simulink library "nexys2iroobo_lib"  (Simulink 7.9)
settings: Solver=ode45  StartTime=0.0  StopTime=10.0  RelTol=1e-3
libraries: xbsIndex_r4 x5
settings Model: Creator=gaborsz  LastModifiedBy=gaborsz

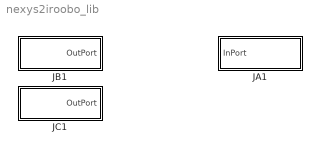
== system nexys2iroobo_lib ==
  JA1 : Subsystem  mask(Non-Memory-Mapped Output Port){show_out=off}
      mask prompts: show_out "Provide Output Double"
      mask help:
      | Port Name: "JA1"
      | Port Type: 8-bit Vector
      mask init:
      | [bg,fg] = xlcmap('IO',0);
      | iPos = get_param(gcb,'Position');
      | iWidth=iPos(3)-iPos(1);
      | iHeight=iPos(4)-iPos(2);
      | [logoX, logoY] = xlogo(iPos);
      | if (show_out)
      |     old = find_system(gcb, 'LookUnderMasks', 'all', 'Name', 'Terminator');
      |     if (length(old) > 0)
      |         replace_block(gcb, 'Name', 'Terminator', 'OutPort', 'noprompt');
      |         set_param([gcb '/Terminator'], 'Name', 'OutPort');
      |     end
      |     portdir = 'output';
      |     portstr = 'dbl';
      | else
      |     old = find_system(gcb, 'LookUnderMasks', 'all', 'name', 'OutPort');
      |     if (length(old) > 0)
      |         replace_block(gcb, 'Name', 'OutPort', 'Terminator', 'noprompt');
      |         set_param([gcb '/OutPort'], 'Name', 'Terminator');
      |     end
      |     portdir = 'input';
      |     portstr = '';
      | end
      settings: CopyFcn=set_param(gcb,'LinkStatus','inactive');
      mask Display:
      | patch([0 iWidth iWidth 0],[0 0 iHeight iHeight] , bg);
      | patch(logoX,logoY, fg);
      | plot([0 0 iWidth iWidth 0], [0 iHeight iHeight 0 0]);
      | port_label(portdir,1,portstr);
      | port_label('input',1,'JA1');
      | text(iWidth-10,5,'nmm');
  JB1 : Subsystem  mask(Non-Memory-Mapped Input Port){signed=off, bpt=0, show_in=off, c=0}
      mask prompts: signed "Signed  (2's comp)"; bpt "Binary Point"; show_in "Provide Input Double"; c "Constant for Simulation"
      mask help:
      | Port Name: "JB1"
      | Port Type: 8-bit Vector
      mask init:
      | [bg,fg] = xlcmap('IO',0);
      | iPos = get_param(gcb,'Position');
      | iWidth=iPos(3)-iPos(1);
      | iHeight=iPos(4)-iPos(2);
      | [logoX, logoY] = xlogo(iPos);
      | if (signed)
      |     set_param([gcb '/JB1'],'arith_type','Signed  (2''s comp)');
      | else
      |     set_param([gcb '/JB1'],'arith_type','Unsigned');
      | end
      | if (show_in)
      |     old = find_system(gcb, 'LookUnderMasks', 'all', 'Name', 'Constant');
      |     if (length(old) > 0)
      |         replace_block(gcb, 'Name', 'Constant', 'InPort', 'noprompt');
      |         set_param([gcb '/Constant'], 'Name', 'InPort');
      |     end
      |     portdir = 'input';
      |     portstr = 'dbl';
      | else
      |     old = find_system(gcb, 'LookUnderMasks', 'all', 'Name', 'InPort');
      |     if (length(old) > 0)
      |         replace_block(gcb, 'Name', 'InPort', 'Constant', 'noprompt');
      |         set_param([gcb '/InPort'], 'Name', 'Constant');
      |         set_param([gcb '/Constant'], 'Value', 'c');
      |     end
      |     portdir = 'output';
      |     portstr = '';
      | end
      settings: CopyFcn=set_param(gcb,'LinkStatus','inactive');
      mask CallbackString:
      | ||mask_vis = get_param(gcb, 'MaskVisibilities');
      | if (strcmp(get_param(gcb, 'show_in'),'on'))
      |     mask_vis(4) = {'off'};
      | else
      |     mask_vis(4) = {'on'};
      | end
      | set_param(gcb, 'MaskVisibilities', mask_vis);
      | |
      mask Display:
      | patch([0 iWidth iWidth 0],[0 0 iHeight iHeight] , bg);
      | patch(logoX,logoY, fg);
      | plot([0 0 iWidth iWidth 0], [0 iHeight iHeight 0 0]);
      | port_label(portdir,1,portstr);
      | port_label('output',1,'JB1');
      | text(2,5,'nmm');
  JC1 : Subsystem  mask(Non-Memory-Mapped Input Port){signed=off, bpt=0, show_in=off, c=0}
      mask prompts: signed "Signed  (2's comp)"; bpt "Binary Point"; show_in "Provide Input Double"; c "Constant for Simulation"
      mask help:
      | Port Name: "JC1"
      | Port Type: 8-bit Vector
      mask init:
      | [bg,fg] = xlcmap('IO',0);
      | iPos = get_param(gcb,'Position');
      | iWidth=iPos(3)-iPos(1);
      | iHeight=iPos(4)-iPos(2);
      | [logoX, logoY] = xlogo(iPos);
      | if (signed)
      |     set_param([gcb '/JC1'],'arith_type','Signed  (2''s comp)');
      | else
      |     set_param([gcb '/JC1'],'arith_type','Unsigned');
      | end
      | if (show_in)
      |     old = find_system(gcb, 'LookUnderMasks', 'all', 'Name', 'Constant');
      |     if (length(old) > 0)
      |         replace_block(gcb, 'Name', 'Constant', 'InPort', 'noprompt');
      |         set_param([gcb '/Constant'], 'Name', 'InPort');
      |     end
      |     portdir = 'input';
      |     portstr = 'dbl';
      | else
      |     old = find_system(gcb, 'LookUnderMasks', 'all', 'Name', 'InPort');
      |     if (length(old) > 0)
      |         replace_block(gcb, 'Name', 'InPort', 'Constant', 'noprompt');
      |         set_param([gcb '/InPort'], 'Name', 'Constant');
      |         set_param([gcb '/Constant'], 'Value', 'c');
      |     end
      |     portdir = 'output';
      |     portstr = '';
      | end
      settings: CopyFcn=set_param(gcb,'LinkStatus','inactive');
      mask CallbackString:
      | ||mask_vis = get_param(gcb, 'MaskVisibilities');
      | if (strcmp(get_param(gcb, 'show_in'),'on'))
      |     mask_vis(4) = {'off'};
      | else
      |     mask_vis(4) = {'on'};
      | end
      | set_param(gcb, 'MaskVisibilities', mask_vis);
      | |
      mask Display:
      | patch([0 iWidth iWidth 0],[0 0 iHeight iHeight] , bg);
      | patch(logoX,logoY, fg);
      | plot([0 0 iWidth iWidth 0], [0 iHeight iHeight 0 0]);
      | port_label(portdir,1,portstr);
      | port_label('output',1,'JC1');
      | text(2,5,'nmm');

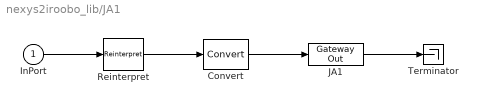
== system nexys2iroobo_lib/JA1 ==
  InPort : Inport
  Convert : xbsIndex_r4/Convert  gui_display_data_type=Fixed-point  arith_type=Unsigned  n_bits=8  bin_pt=0  float_type=Single  exp_bits=8  fraction_bits=24  quantization=Truncate  overflow=Wrap  en=off  latency=0  dbl_ovrd=off  pipeline=off  block_type=convert
  JA1 : xbsIndex_r4/Gateway Out  inherit_from_input=off  hdl_port=on  timing_constraint=None  locs_specified=on  LOCs={'M16','M14','L16','K13','M15','L17','K12','L15'}  UseAsDAC=off  DACChannel='1'  block_type=gatewayout
      settings: sginterface={'Xilinx'=>{'jtaghwcosim'=>{'non_memory_mapped_port'=>'JA1'}}}
  Reinterpret : xbsIndex_r4/Reinterpret  force_arith_type=off  arith_type=Unsigned  force_bin_pt=off  bin_pt=0  block_type=reinterpret
  Terminator : Terminator
  wires:
  InPort/1 -> Reinterpret/1
  Reinterpret/1 -> Convert/1
  Convert/1 -> JA1/1
  JA1/1 -> Terminator/1

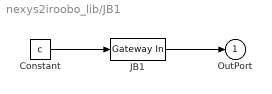
== system nexys2iroobo_lib/JB1 ==
  Constant : Constant  Value=c
  JB1 : xbsIndex_r4/Gateway In  gui_display_data_type=Fixed-point  arith_type=Unsigned  n_bits=8  bin_pt=max(0,min(bpt,8))  preci_type=Single  exp_width=8  frac_width=24  quantization="Round  (unbiased: +/- Inf)"  overflow=Saturate  period=1  dbl_ovrd=off  timing_constraint=None  locs_specified=on  LOCs={'U18','T18','R16','P17','T17','R15','R18','M13'}  UseAsADC=off  ADCChannel='1'  inherit_from_input=off  hdl_port=on  block_type=gatewayin
      settings: sginterface={'Xilinx'=>{'jtaghwcosim'=>{'non_memory_mapped_port'=>'JB1'}}}
  OutPort : Outport
  wires:
  Constant/1 -> JB1/1
  JB1/1 -> OutPort/1

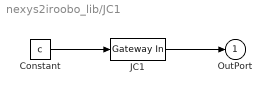
== system nexys2iroobo_lib/JC1 ==
  Constant : Constant  Value=c
  JC1 : xbsIndex_r4/Gateway In  gui_display_data_type=Fixed-point  arith_type=Unsigned  n_bits=8  bin_pt=max(0,min(bpt,8))  preci_type=Single  exp_width=8  frac_width=24  quantization="Round  (unbiased: +/- Inf)"  overflow=Saturate  period=1  dbl_ovrd=off  timing_constraint=None  locs_specified=on  LOCs={'J12','G16','F14','H15','H16','G13','J16','G15'}  UseAsADC=off  ADCChannel='1'  inherit_from_input=off  hdl_port=on  block_type=gatewayin
      settings: sginterface={'Xilinx'=>{'jtaghwcosim'=>{'non_memory_mapped_port'=>'JC1'}}}
  OutPort : Outport
  wires:
  Constant/1 -> JC1/1
  JC1/1 -> OutPort/1
